simulink model "rigid_body_dynamics_discrete"  (R2020b)
settings: Solver=VariableStepAuto  StartTime=0.0  StopTime=10.0  RelTol=1e-3
values from neighbouring files (symbols this model uses):
  SampleTime = 0.001    [iris_quadcopter_specs.m]
undefined symbols (not defined in the file or in its folder): DiscIntNeverNeededParam
libraries: shared6dof x4, shared6dofsys x3, sharedutil x1
settings Model: Creator=sid  LastModifiedBy=sid

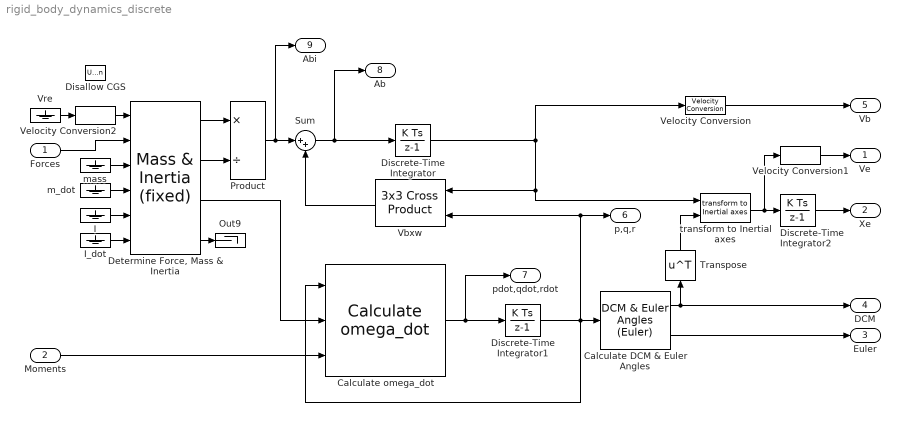
== system rigid_body_dynamics_discrete ==
  Forces : Inport  Unit=N  PortDimensions=3
  Moments : Inport  Port=2  Unit=N*m  PortDimensions=3
  Calculate DCM & Euler Angles : shared6dofsys/DCM & Euler Angles (Euler)  aMode=aMode
      settings: SourceProductBaseCode=AE,PW,MT,UV,VE,VP
  Calculate omega_dot : shared6dofsys/Calculate omega_dot  aMode=aMode
      settings: SourceProductBaseCode=AE,PW,MT,UV,VE,VP
  "Determine Force, Mass & Inertia" : shared6dofsys/Mass & Inertia (fixed)  aMode=aMode
      settings: SourceProductBaseCode=AE,PW,MT,UV,VE,VP
  Disallow CGS : UnitConfiguration  UnitSystemsStr=English,SI,SI (extended)  AllowAllUnitSystems=off
  Discrete-Time Integrator : DiscreteIntegrator  SampleTime=SampleTime  ICPrevOutput=DiscIntNeverNeededParam  ICPrevScaledInput=DiscIntNeverNeededParam
  Discrete-Time Integrator1 : DiscreteIntegrator  SampleTime=SampleTime  ICPrevOutput=DiscIntNeverNeededParam  ICPrevScaledInput=DiscIntNeverNeededParam
  Discrete-Time Integrator2 : DiscreteIntegrator  SampleTime=SampleTime  ICPrevOutput=DiscIntNeverNeededParam  ICPrevScaledInput=DiscIntNeverNeededParam
  I : Ground
  I_dot : Ground
  Out9 : Terminator
  Product : Product  Inputs=*/  SaturateOnIntegerOverflow=on  OutDataTypeStr=Inherit: Same as first input
  Sum : Sum  Inputs=|++  SaturateOnIntegerOverflow=on
  Transpose : Math  Operator=transpose  SignedPower=on  SaturateOnIntegerOverflow=on
  Vbxw : sharedutil/3x3 Cross Product  aMode=aMode
      settings: SourceProductBaseCode=AE,PW,MT,UV,VE,VP
  Velocity Conversion : shared6dof/6DOF (Euler Angles)/Velocity Conversion  SystemSampleTime=-1  VariantActivationTime=update diagram  Latency=0  AutoFrameSizeCalculation=off
      settings: SourceProductBaseCode=AE,PW,MT,UV,VE,VP
  Velocity Conversion1 : shared6dof/6DOF (Euler Angles)/Velocity Conversion1  SystemSampleTime=-1  VariantActivationTime=update diagram  Latency=0  AutoFrameSizeCalculation=off
      settings: SourceProductBaseCode=AE,PW,MT,UV,VE,VP
  Velocity Conversion2 : shared6dof/6DOF (Euler Angles)/Velocity Conversion2  SystemSampleTime=-1  VariantActivationTime=update diagram  Latency=0  AutoFrameSizeCalculation=off
      settings: SourceProductBaseCode=AE,PW,MT,UV,VE,VP
  Vre : Ground
  m_dot : Ground
  mass : Ground
  "transform to Inertial axes " : shared6dof/6DOF (Euler Angles)/transform to Inertial axes   SystemSampleTime=-1  VariantActivationTime=update diagram  Latency=0  AutoFrameSizeCalculation=off
      settings: SourceProductBaseCode=AE,PW,MT,UV,VE,VP
  Ve : Outport  Unit=m/s  VectorParamsAs1DForOutWhenUnconnected=off
  Xe : Outport  Port=2  Unit=m  VectorParamsAs1DForOutWhenUnconnected=off
  Euler : Outport  Port=3  Unit=rad  VectorParamsAs1DForOutWhenUnconnected=off
  DCM : Outport  Port=4  Unit=1  VectorParamsAs1DForOutWhenUnconnected=off
  Vb : Outport  Port=5  Unit=m/s  VectorParamsAs1DForOutWhenUnconnected=off
  p,q,r : Outport  Port=6  Unit=rad/s  VectorParamsAs1DForOutWhenUnconnected=off
  pdot,qdot,rdot : Outport  Port=7  Unit=rad/s^2  VectorParamsAs1DForOutWhenUnconnected=off
  Ab : Outport  Port=8  Unit=m/s^2  VectorParamsAs1DForOutWhenUnconnected=off
  Abi : Outport  Port=9  Unit=m/s^2
  wires:
  Discrete-Time Integrator2/1 -> Xe/1
  Discrete-Time Integrator/1 -> "transform to Inertial axes "/1, Vbxw/1, Velocity Conversion/1
  Velocity Conversion1/1 -> Ve/1
  Vre/1 -> Velocity Conversion2/1
  Moments/1 -> Calculate omega_dot/3
  Calculate DCM & Euler Angles/1 -> Transpose/1, DCM/1
  Vbxw/1 -> Sum/2
  mass/1 -> "Determine Force, Mass & Inertia"/3
  Product/1 -> Sum/1, Abi/1
  Discrete-Time Integrator1/1 -> Calculate DCM & Euler Angles/1, Calculate omega_dot/1, p,q,r/1, Vbxw/2
  Calculate omega_dot/1 -> Discrete-Time Integrator1/1, pdot,qdot,rdot/1
  I/1 -> "Determine Force, Mass & Inertia"/5
  "Determine Force, Mass & Inertia"/4 -> Out9/1
  "Determine Force, Mass & Inertia"/1 -> Product/1
  Velocity Conversion2/1 -> "Determine Force, Mass & Inertia"/1
  Transpose/1 -> "transform to Inertial axes "/2
  Velocity Conversion/1 -> Vb/1
  "transform to Inertial axes "/1 -> Velocity Conversion1/1, Discrete-Time Integrator2/1
  "Determine Force, Mass & Inertia"/2 -> Product/2
  Sum/1 -> Discrete-Time Integrator/1, Ab/1
  "Determine Force, Mass & Inertia"/3 -> Calculate omega_dot/2
  Forces/1 -> "Determine Force, Mass & Inertia"/2
  Calculate DCM & Euler Angles/2 -> Euler/1
  I_dot/1 -> "Determine Force, Mass & Inertia"/6
  m_dot/1 -> "Determine Force, Mass & Inertia"/4
